simulink model "labSim"  (R2019a)
settings: Solver=VariableStepAuto  StartTime=0.0  StopTime=10.0  RelTol=1e-3
settings Model: Creator=G5  LastModifiedBy=G5

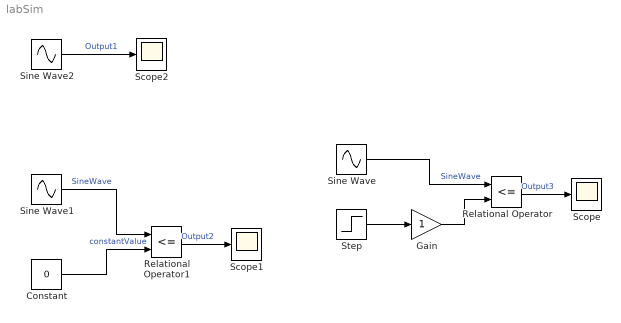
== system labSim ==
  Constant : Constant  Value=0
  Gain : Gain
  Relational Operator : RelationalOperator  Operator=<=  OutDataTypeStr=boolean  RndMeth=Simplest
  Relational Operator1 : RelationalOperator  Operator=<=  OutDataTypeStr=boolean  RndMeth=Simplest
  Scope : Scope
  Scope1 : Scope
  Scope2 : Scope
  Sine Wave : Sin  SampleTime=0
  Sine Wave1 : Sin  SampleTime=0
  Sine Wave2 : Sin  SampleTime=0
  Step : Step  Time=2  SampleTime=0
  wires:
  Relational Operator/1 -> Scope/1  "Output3"
  Step/1 -> Gain/1
  Gain/1 -> Relational Operator/2
  Sine Wave/1 -> Relational Operator/1  "SineWave"
  Constant/1 -> Relational Operator1/2  "constantValue"
  Sine Wave1/1 -> Relational Operator1/1  "SineWave"
  Relational Operator1/1 -> Scope1/1  "Output2"
  Sine Wave2/1 -> Scope2/1  "Output1"
